simulink model "IRp-6"  (R2021b)
settings: Solver=ode1  StartTime=0.0  StopTime=Inf  FixedStep=0.001  RelTol=1e-3  EnableMultiTasking=on
PostLoadFcn:
  | , if any(exist('dsrtsu_mdlpostloadfcn', 'file') == [2, 3, 6]), try dsrtsu_mdlpostloadfcn('Execute', bdroot); catch fprintf('Error in PostLoadFcn (dsrtsu_mdlpostloadfcn) for model "%s":\n %s\n', bdroot, lasterr); end, end,
libraries: rtilibm x3
(part 2 of 2)

== system IRp-6/Position 3/Filters 3/Analog Butterworth LP Filter ==
  In1 : Inport
  Analog Butterworth LP Filter : ZeroPole  Zeros=z  Poles=p  Gain=k
  Out1 : Outport
  wires:
  In1/1 -> Analog Butterworth LP Filter/1
  Analog Butterworth LP Filter/1 -> Out1/1

== system IRp-6/Position 3/Filters 3/Analog Butterworth LP Filter1 ==
  In1 : Inport
  Analog Butterworth LP Filter1 : ZeroPole  Zeros=z  Poles=p  Gain=k
  Out1 : Outport
  wires:
  In1/1 -> Analog Butterworth LP Filter1/1
  Analog Butterworth LP Filter1/1 -> Out1/1

== system IRp-6/Position 4/Filters 4/Analog Butterworth LP Filter ==
  In1 : Inport
  Analog Butterworth LP Filter : ZeroPole  Zeros=z  Poles=p  Gain=k
  Out1 : Outport
  wires:
  In1/1 -> Analog Butterworth LP Filter/1
  Analog Butterworth LP Filter/1 -> Out1/1

== system IRp-6/Position 4/Filters 4/Analog Butterworth LP Filter1 ==
  In1 : Inport
  Analog Butterworth LP Filter1 : ZeroPole  Zeros=z  Poles=p  Gain=k
  Out1 : Outport
  wires:
  In1/1 -> Analog Butterworth LP Filter1/1
  Analog Butterworth LP Filter1/1 -> Out1/1

== system IRp-6/Position 5/Filters 5/Analog Butterworth LP Filter ==
  In1 : Inport
  Analog Butterworth LP Filter : ZeroPole  Zeros=z  Poles=p  Gain=k
  Out1 : Outport
  wires:
  In1/1 -> Analog Butterworth LP Filter/1
  Analog Butterworth LP Filter/1 -> Out1/1

== system IRp-6/Position 5/Filters 5/Analog Butterworth LP Filter1 ==
  In1 : Inport
  Analog Butterworth LP Filter1 : ZeroPole  Zeros=z  Poles=p  Gain=k
  Out1 : Outport
  wires:
  In1/1 -> Analog Butterworth LP Filter1/1
  Analog Butterworth LP Filter1/1 -> Out1/1

== system IRp-6/RTI Data/RTI Data Store/RTI Data Store ==
  RTI Data Store : Subsystem  mask(RTI_DATA_STORE){}
      mask help:
      | RTI Data Store Block. This block is used by RTI to store internal model dependent data. Deleting this block will result in data loss.
      |
      | NEVER DELETE, COPY, OR MODIFY THIS BLOCK!
      mask Help:
      | RTI Data Store Block. This block is used by RTI to store internal model dependent data. Deleting this block will result in data loss.
      | 
      | NEVER DELETE, COPY, OR MODIFY THIS BLOCK!
      mask Display: text(0.5, 0.5, ' ', 'HorizontalAlignment', 'center');

== system IRp-6/RTI Data/RTI Data Store/RTI Data Store/RTI Data Store ==
  RTI Data Store : Subsystem  mask(RTI_DATA_STORE){}
      mask help:
      | RTI Data Store Block. This block is used by RTI to store internal model dependent data. Deleting this block will result in data loss.
      |
      | NEVER DELETE, COPY, OR MODIFY THIS BLOCK!
      mask Help:
      | RTI Data Store Block. This block is used by RTI to store internal model dependent data. Deleting this block will result in data loss.
      | 
      | NEVER DELETE, COPY, OR MODIFY THIS BLOCK!
      mask Display: text(0.5, 0.5, ' ', 'HorizontalAlignment', 'center');

== system IRp-6/RTI Data/RTI Data Store/RTI Data Store/RTI Data Store/RTI Data Store ==

== matlab function IRp-6/Serwo 3/Wybór pomiędzy bazowaniem a pracą normalną ==
  data: baz input; y output; czuj input; res output; ster input
function [y, res] = fcn(baz, czuj, ster)
if baz && ~czuj
    y = -0.3;
    res = 0;
else
    y = ster;
    res = 1;
end

== matlab function IRp-6/Synchronizacja ramion robota ==
  data: trybs input; trybw input; wyzw input; wym1 input; wym2 input; wym3 input; v1 output; poz1 input; poz2 input; poz3 input; v2 output; v3 output; memo1 input; memo2 input; memo3 input
function [v1, v2, v3] = fcn(trybs, trybw, wyzw, wym1, wym2, wym3, poz1, poz2, poz3, memo1, memo2, memo3)
% Wyliczanie synchronizacji prędkości przed wyzwoleniem
if trybs && trybw && ~wyzw
    angle1 = abs(wym1-poz1);
    angle2 = abs(wym2-poz2);
    angle3 = abs(wym3-poz3);
    if angle1 >= angle2 && angle1 >= angle3
        v1 = 1;
        v2 = angle2/angle1;
        v3 = angle3/angle1;
    elseif angle2 >= angle1 && angle2 >= angle3
        v1 = angle1/angle2;
        v2 = 1;
        v3 = angle3/angle2;
    elseif angle3 >= angle1 && angle3 >= angle2
        v1 = angle1/angle3;
        v2 = angle2/angle3;
        v3 = 1;
    else
        v1 = 1;
        v2 = 1;
        v3 = 1;
    end
% Podtrzymanie wyliczonych prędkości po wyzwoleniu
elseif trybs && trybw && wyzw
    v1 = memo1;
    v2 = memo2;
    v3 = memo3;
% Nieuwzględnianie synchronizacji przy trybie "pracy ręcznej" oraz przy
% wyłączonym trybie PTP Synchronicznym
else
    v1 = 1;
    v2 = 1;
    v3 = 1;
end

== matlab function IRp-6/Zadanie kinematyki prostej ==
  data: dx output; pos1 input; pos2 input; pos3 input; dy output; dz output
function [dx, dy, dz] = fcn(pos1, pos2, pos3)
% Przeliczenie kątów na radiany
phi1 = pos1 * pi / 180;
phi2 = pos2 * pi / 180;
phi3 = pos3 * pi / 180;
% Długości ramion robota w [mm]
p1 = 700;
p2 = 450;
p3 = 670;
% Wyliczenie pozycji końcówki w przestrzeni kartezjańskiej
% Jednostka ta sama co przy długościach ramion robota
dx = cos(phi1) * (p3*cos(-phi3) + p2*cos(pi/2-phi2));
dy = sin(phi1) * (p3*cos(-phi3) + p2*cos(pi/2-phi2));
dz = p3*sin(-phi3) + p2*sin(pi/2-phi2) + p1;

== matlab function IRp-6/Serwo 1/Obsługa trybu pracy ==
  data: ster input; tryb input; wyzw input; memo input; y output
function y = fcn(ster, tryb, wyzw, memo)
% Tryb "pracy ręcznej"
if ~tryb
    y = ster;
% Tryb "wyzwalany"
else
    if ~wyzw
        y = memo;
    else
        y = ster;
    end
end

== matlab function IRp-6/Serwo 1/Zerowanie wymuszenia po zbazowaniu ==
  data: wym input; baz input; y output; czuj input
function y = fcn(wym, baz, czuj)
if baz && czuj
   y =  0;
else
    y = wym;
end

== matlab function IRp-6/Serwo 1/Wybór pomiędzy bazowaniem a pracą normalną ==
  data: baz input; y output; czuj input; res output; ster input
function [y, res] = fcn(baz, czuj, ster)
if baz && ~czuj
    y = -0.3;
    res = 0;
else
    y = ster;
    res = 1;
end

== matlab function IRp-6/Serwo 1/Zadanie prędkości ==
  data: ster input; pred input; y output
function y = fcn(ster, pred)
if pred >= 1 && pred <= 100
    y = ster*pred/100;
else
    y = ster;
end

== matlab function IRp-6/Serwo 2/Zadanie prędkości ==
  data: ster input; pred input; y output
function y = fcn(ster, pred)
if pred >= 1 && pred <= 100
    y = ster*pred/100;
else
    y = ster;
end

== matlab function IRp-6/Serwo 2/Zerowanie wymuszenia po zbazowaniu ==
  data: wym input; baz input; y output; czuj input
function y = fcn(wym, baz, czuj)
if baz && czuj
   y =  0;
else
    y = wym;
end

== matlab function IRp-6/Serwo 3/Zadanie prędkości ==
  data: ster input; pred input; y output
function y = fcn(ster, pred)
if pred >= 1 && pred <= 100
    y = ster*pred/100;
else
    y = ster;
end

== matlab function IRp-6/Wyłącznik wyzwalania ==
  data: tryb input; wyzw input; wym1 input; wym2 input; wym3 input; y output; poz1 input; poz2 input; poz3 input
function y = fcn(tryb, wyzw, wym1, wym2, wym3, poz1, poz2, poz3)
eps = 1;
if tryb && wyzw && abs(wym1-poz1) <= eps && abs(wym2-poz2) <= eps && abs(wym3-poz3) <= eps
    y = 0;
else
    y = wyzw;
end

== matlab function IRp-6/Serwo 3/Zerowanie wymuszenia po zbazowaniu ==
  data: wym input; baz input; y output; czuj input
function y = fcn(wym, baz, czuj)
if baz && czuj
   y =  0;
else
    y = wym;
end

== matlab function IRp-6/Serwo 2/Obsługa trybu pracy ==
  data: ster input; tryb input; wyzw input; memo input; y output
function y = fcn(ster, tryb, wyzw, memo)
% Tryb "pracy ręcznej"
if ~tryb
    y = ster;
% Tryb "wyzwalany"
else
    if ~wyzw
        y = memo;
    else
        y = ster;
    end
end

== matlab function IRp-6/Serwo 1/Sprawdzanie ograniczeń ==
  data: wym input; memo input; y output
function y = fcn(wym, memo)
if wym > -160 && wym < 160
        y = wym;
else
        y = memo;
end

== matlab function IRp-6/Wyłącznik bazowania ==
  data: baz input; y output; czuj1 input; czuj2 input; czuj3 input; wym1 input; wym2 input; wym3 input
function y = fcn(baz, czuj1, czuj2, czuj3, wym1, wym2, wym3)
if baz && czuj1 && czuj2 && czuj3 && ~wym1 && ~wym2 && ~wym3
   y =  0;
else
    y = baz;
end

== matlab function IRp-6/Serwo 2/Sprawdzanie ograniczeń ==
  data: wym input; phi input; memo input; y output
function y = fcn(wym, phi, memo)
if wym > -40 && wym < 40 && abs(wym-phi) <= 40
        y = wym;
else
        y = memo;
end

== matlab function IRp-6/Serwo 2/Wybór pomiędzy bazowaniem a pracą normalną ==
  data: baz input; y output; czuj input; res output; ster input
function [y, res] = fcn(baz, czuj, ster)
if baz && ~czuj
    y = -0.3;
    res = 0;
else
    y = ster;
    res = 1;
end

== matlab function IRp-6/Serwo 3/Obsługa trybu pracy ==
  data: ster input; tryb input; wyzw input; memo input; y output
function y = fcn(ster, tryb, wyzw, memo)
% Tryb "pracy ręcznej"
if ~tryb
    y = ster;
% Tryb "wyzwalany"
else
    if ~wyzw
        y = memo;
    else
        y = ster;
    end
end

== matlab function IRp-6/Serwo 3/Sprawdzanie ograniczeń ==
  data: wym input; phi input; memo input; y output
function y = fcn(wym, phi, memo)
if wym > -40 && wym < 40 && abs(wym-phi) <= 40
        y = wym;
else
        y = memo;
end
